simulink model "models4"  (R2020a)
settings: Solver=FixedStepAuto  StartTime=0.0  StopTime=0.3  FixedStep=1e-4  RelTol=1e-3
settings Model: Creator=denim  LastModifiedBy=denim

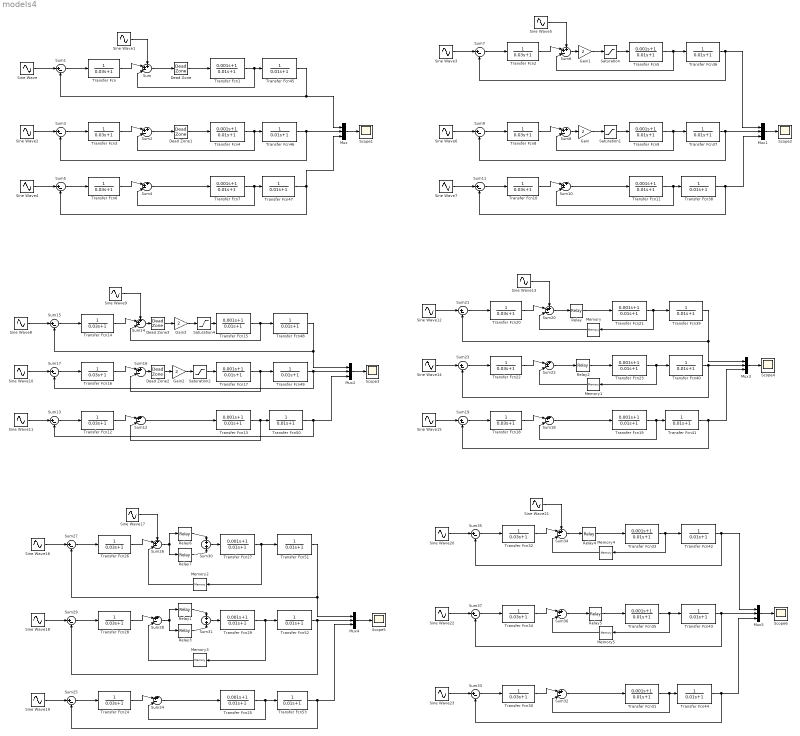
== system models4 ==
  Dead Zone{,1..3} (4 alike) : DeadZone  LowerValue=-1  UpperValue=1  SaturateOnIntegerOverflow=on
  Gain{,1..3} (4 alike) : Gain  Gain=2
  Memory{,1..5} (6 alike) : Memory
  Mux{,1..5} (6 alike) : Mux  Inputs=3
  Relay : Relay  OnSwitchValue=0  OffSwitchValue=0  OnOutputValue=2  OffOutputValue=-2
  Relay1 : Relay  OnSwitchValue=-1  OffSwitchValue=-1  OnOutputValue=0  OffOutputValue=-2
  Relay2 : Relay  OnSwitchValue=0  OffSwitchValue=0  OnOutputValue=2  OffOutputValue=-2
  Relay3 : Relay  OnSwitchValue=1  OffSwitchValue=1  OnOutputValue=2
  Relay4 : Relay  OnSwitchValue=1  OffSwitchValue=-1  OnOutputValue=2  OffOutputValue=-2
  Relay5 : Relay  OnSwitchValue=1  OffSwitchValue=-1  OnOutputValue=2  OffOutputValue=-2
  Relay6 : Relay  OnSwitchValue=-1  OffSwitchValue=-1  OnOutputValue=0  OffOutputValue=-2
  Relay7 : Relay  OnSwitchValue=1  OffSwitchValue=1  OnOutputValue=2
  Saturation : Saturate  UpperLimit=1  LowerLimit=-1
  Saturation1 : Saturate  UpperLimit=1  LowerLimit=-1
  Saturation2 : Saturate  UpperLimit=2  LowerLimit=-2
  Saturation4 : Saturate  UpperLimit=2  LowerLimit=-2
  Scope{1..6} (6 alike) : Scope
  Sine Wave{,2..4,6..8,10..12,14..16,18..20,22..23} (18 alike) : Sin  Amplitude=4  Frequency=150  SampleTime=0
  Sine Wave1 : Sin  Amplitude=6  Frequency=1500  SampleTime=0
  Sine Wave13 : Sin  Amplitude=1.5  Frequency=1500  SampleTime=0
  Sine Wave17 : Sin  Amplitude=1.9  Frequency=1500  SampleTime=0
  Sine Wave21 : Sin  Amplitude=1.6  Frequency=1500  SampleTime=0
  Sine Wave5 : Sin  Amplitude=0.9  Frequency=1500  SampleTime=0
  Sine Wave9 : Sin  Amplitude=2.9  Frequency=1500  SampleTime=0
  Sum{,2,4,6,8,10,12,14,16,18,20,22,24,26,28,32,34,36} (18 alike) : Sum  Inputs=++-|
  Sum{1,3,5,7,9,11,13,15,17,19,21,23,25,27,29,33,35,37} (18 alike) : Sum  Inputs=|+-
  Sum30 : Sum
  Sum31 : Sum
  Transfer Fcn{,2..3,6,8,10,12,14,16,18,20,22,24,26,28,30,32,34} (18 alike) : TransferFcn  Denominator=[0.03 1]
  Transfer Fcn{1,4..5,7,9,11,13,15,17,19,21,23,25,27,29,31,33,35} (18 alike) : TransferFcn  Numerator=[0.001 1]  Denominator=[0.01 1]
  Transfer Fcn{36..53} (18 alike) : TransferFcn  Denominator=[0.01 1]
  wires:
  Sum1/1 -> Transfer Fcn/1
  Sum/1 -> Dead Zone/1
  Transfer Fcn1/1 -> Transfer Fcn45/1, Sum/3
  Transfer Fcn45/1 -> Mux/1, Sum1/2
  Transfer Fcn/1 -> Sum/2
  Sine Wave/1 -> Sum1/1
  Sine Wave1/1 -> Sum/1
  Sine Wave2/1 -> Sum3/1
  Dead Zone1/1 -> Transfer Fcn4/1
  Transfer Fcn4/1 -> Transfer Fcn46/1, Sum2/3
  Sum2/1 -> Dead Zone1/1
  Sum3/1 -> Transfer Fcn3/1
  Transfer Fcn46/1 -> Mux/2, Sum3/2
  Transfer Fcn3/1 -> Sum2/2
  Sine Wave4/1 -> Sum5/1
  Transfer Fcn7/1 -> Transfer Fcn47/1, Sum4/3
  Sum5/1 -> Transfer Fcn6/1
  Transfer Fcn47/1 -> Mux/3, Sum5/2
  Transfer Fcn6/1 -> Sum4/2
  Sum4/1 -> Transfer Fcn7/1
  Dead Zone/1 -> Transfer Fcn1/1
  Mux/1 -> Scope1/1
  Saturation1/1 -> Transfer Fcn9/1
  Sine Wave3/1 -> Sum7/1
  Transfer Fcn38/1 -> Mux1/3, Sum11/2
  Transfer Fcn10/1 -> Sum10/2
  Transfer Fcn9/1 -> Transfer Fcn37/1, Sum8/3
  Sum11/1 -> Transfer Fcn10/1
  Transfer Fcn11/1 -> Transfer Fcn38/1, Sum10/3
  Sine Wave7/1 -> Sum11/1
  Sine Wave6/1 -> Sum9/1
  Sine Wave5/1 -> Sum6/1
  Sum10/1 -> Transfer Fcn11/1
  Transfer Fcn5/1 -> Transfer Fcn36/1, Sum6/3
  Saturation/1 -> Transfer Fcn5/1
  Transfer Fcn8/1 -> Sum8/2
  Sum9/1 -> Transfer Fcn8/1
  Transfer Fcn36/1 -> Mux1/1, Sum7/2
  Sum7/1 -> Transfer Fcn2/1
  Mux1/1 -> Scope2/1
  Transfer Fcn2/1 -> Sum6/2
  Transfer Fcn37/1 -> Mux1/2, Sum9/2
  Sum6/1 -> Gain1/1
  Sum8/1 -> Gain/1
  Transfer Fcn14/1 -> Sum14/2
  Mux2/1 -> Scope3/1
  Transfer Fcn49/1 -> Mux2/2, Sum17/2
  Sum15/1 -> Transfer Fcn14/1
  Sum17/1 -> Transfer Fcn16/1
  Sine Wave8/1 -> Sum15/1
  Sine Wave11/1 -> Sum13/1
  Transfer Fcn16/1 -> Sum16/2
  Transfer Fcn48/1 -> Mux2/1, Sum15/2
  Transfer Fcn15/1 -> Transfer Fcn48/1, Sum14/3
  Sine Wave9/1 -> Sum14/1
  Sine Wave10/1 -> Sum17/1
  Sum12/1 -> Transfer Fcn13/1
  Sum13/1 -> Transfer Fcn12/1
  Transfer Fcn50/1 -> Mux2/3, Sum13/2
  Transfer Fcn12/1 -> Sum12/2
  Transfer Fcn13/1 -> Transfer Fcn50/1, Sum12/3
  Transfer Fcn17/1 -> Transfer Fcn49/1, Sum16/3
  Dead Zone3/1 -> Gain3/1
  Sum14/1 -> Dead Zone3/1
  Saturation4/1 -> Transfer Fcn15/1
  Dead Zone2/1 -> Gain2/1
  Sum16/1 -> Dead Zone2/1
  Saturation2/1 -> Transfer Fcn17/1
  Transfer Fcn20/1 -> Sum20/2
  Sum22/1 -> Relay2/1
  Mux3/1 -> Scope4/1
  Transfer Fcn40/1 -> Mux3/2, Sum23/2
  Sum21/1 -> Transfer Fcn20/1
  Sum23/1 -> Transfer Fcn22/1
  Sine Wave12/1 -> Sum21/1
  Sine Wave15/1 -> Sum19/1
  Transfer Fcn22/1 -> Sum22/2
  Transfer Fcn39/1 -> Sum21/2, Mux3/1
  Transfer Fcn21/1 -> Transfer Fcn39/1, Memory/1
  Sine Wave14/1 -> Sum23/1
  Sum18/1 -> Transfer Fcn19/1
  Relay2/1 -> Transfer Fcn23/1
  Sum19/1 -> Transfer Fcn18/1
  Transfer Fcn41/1 -> Mux3/3, Sum19/2
  Transfer Fcn18/1 -> Sum18/2
  Transfer Fcn23/1 -> Transfer Fcn40/1, Memory1/1
  Sine Wave13/1 -> Sum20/1
  Sum20/1 -> Relay/1
  Relay/1 -> Transfer Fcn21/1
  Memory/1 -> Sum20/3
  Memory1/1 -> Sum22/3
  Transfer Fcn19/1 -> Transfer Fcn41/1, Sum18/3
  Mux4/1 -> Scope5/1
  Transfer Fcn51/1 -> Sum27/2, Mux4/1
  Sine Wave19/1 -> Sum25/1
  Transfer Fcn28/1 -> Sum28/2
  Sum29/1 -> Transfer Fcn28/1
  Sine Wave16/1 -> Sum27/1
  Sum25/1 -> Transfer Fcn24/1
  Sum24/1 -> Transfer Fcn25/1
  Transfer Fcn27/1 -> Transfer Fcn51/1, Memory2/1
  Transfer Fcn25/1 -> Transfer Fcn53/1, Sum24/3
  Transfer Fcn29/1 -> Transfer Fcn52/1, Memory3/1
  Memory2/1 -> Sum26/3
  Transfer Fcn24/1 -> Sum24/2
  Transfer Fcn26/1 -> Sum26/2
  Sine Wave18/1 -> Sum29/1
  Transfer Fcn53/1 -> Mux4/3, Sum25/2
  Sum27/1 -> Transfer Fcn26/1
  Sine Wave17/1 -> Sum26/1
  Transfer Fcn52/1 -> Mux4/2, Sum29/2
  Memory3/1 -> Sum28/3
  Sum31/1 -> Transfer Fcn29/1
  Sum30/1 -> Transfer Fcn27/1
  Relay7/1 -> Sum30/2
  Relay6/1 -> Sum30/1
  Sum26/1 -> Relay7/1, Relay6/1
  Relay3/1 -> Sum31/2
  Sum28/1 -> Relay3/1, Relay1/1
  Relay1/1 -> Sum31/1
  Mux5/1 -> Scope6/1
  Transfer Fcn42/1 -> Sum35/2, Mux5/1
  Sine Wave23/1 -> Sum33/1
  Transfer Fcn34/1 -> Sum36/2
  Sum37/1 -> Transfer Fcn34/1
  Sine Wave20/1 -> Sum35/1
  Sum33/1 -> Transfer Fcn30/1
  Sum32/1 -> Transfer Fcn31/1
  Transfer Fcn33/1 -> Transfer Fcn42/1, Memory4/1
  Transfer Fcn31/1 -> Transfer Fcn44/1, Sum32/3
  Transfer Fcn35/1 -> Transfer Fcn43/1, Memory5/1
  Sum34/1 -> Relay4/1
  Memory4/1 -> Sum34/3
  Transfer Fcn30/1 -> Sum32/2
  Transfer Fcn32/1 -> Sum34/2
  Sine Wave22/1 -> Sum37/1
  Transfer Fcn44/1 -> Mux5/3, Sum33/2
  Sum35/1 -> Transfer Fcn32/1
  Sine Wave21/1 -> Sum34/1
  Transfer Fcn43/1 -> Mux5/2, Sum37/2
  Memory5/1 -> Sum36/3
  Relay5/1 -> Transfer Fcn35/1
  Sum36/1 -> Relay5/1
  Relay4/1 -> Transfer Fcn33/1
  Gain1/1 -> Saturation/1
  Gain/1 -> Saturation1/1
  Gain3/1 -> Saturation4/1
  Gain2/1 -> Saturation2/1
